simulink model "testPacketSend"  (R2014a)
settings: Solver=FixedStepDiscrete  StartTime=0.0  StopTime=Inf  FixedStep=0.001  RelTol=1e-3
InitFcn:
  | testSerializedParams_Initialize();
undefined symbols (not defined in the file or in its folder): macaddr
libraries: xpcnetworkbufferlib x1, xpcethernetlib x1, libButtons x1, libBusSerialize x1
settings Model: xpc_rtwmakecfg_data=_xpcnblib__xpcetherlib__xpcether8255xlib__xpcetherGbElib_  SimulationMode=external  BufferReuse=off  Creator=shenoylab  LastModifiedBy=shenoylab
settings SolverCC: EnableConcurrentExecution=on
settings DataIOCC: SignalLoggingSaveFormat=ModelDataLogs
settings OptimizationCC: BlockReduction=off  OptimizeBlockIOStorage=off  BufferReuse=off  GlobalBufferReuse=off  ExpressionFolding=off  LocalBlockOutputs=off
settings DebuggingCC: SaveWithDisabledLinksMsg=none  MultiTaskDSMMsg=warning  MultiTaskCondExecSysMsg=none  StateNameClashWarn=warning
settings HardwareCC: ProdIntDivRoundTo=Zero  ProdEndianess=LittleEndian  ProdHWDeviceType=Generic->32-bit x86 compatible
settings RTWCC: SystemTargetFile=slrt.tlc  TemplateMakefile=slrt_default_tmf  Description=Simulink Real-Time  GenerateReport=on  ProcessScript=slrt_make_rtw_hook  LaunchReport=on  IncludeERTFirstTime=on  RTWCompilerOptimization=On
settings CodeAppCC: MATLABSourceComments=on
settings SimulinkRealTimeCC: GeneratePreprocessorConditionals=Disable all  EnableShiftOperators=on  xpcDblBuff=on

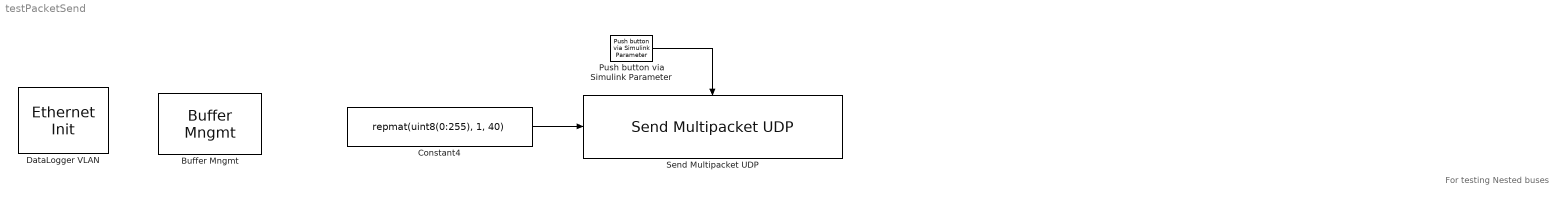
== system testPacketSend ==
  note: For testing Nested buses
  "Buffer Mngmt " : xpcnetworkbufferlib/Buffer Mngmt   Priority=-1  SampleTime=-1  PoolSizes=[256 512 1024 2048]  ShowTune=off
  Constant4 : Constant  Value=repmat(uint8(0:255), 1, 40)
  DataLogger VLAN : xpcethernetlib/Ethernet Init   Priority=-1  ID=2  Driver=Intel 8255x  Bus=3  Slot=5  SampleTime=-1  AddressSource=EEPROM  MAC=macaddr('00:00:00:00:00:00')  TxSA=off  RxPromiscuous=off  Multicast={}  RxBad=off  RxShort=off  MaxMTU=1518  TxThreshold=224  TxBuffers=256  RxBuffers=64  ShowTune=off  NumRxBlks=1
  Push button via Simulink Parameter : libButtons/Push button via Simulink Parameter  paramName='paramtestSerializedParamsExtern0x2FPushButtonViaSimulinkParamet'  Ts=0.001
  Send Multipacket UDP : libBusSerialize/Send Multipacket UDP  transmitId=2  sourceIP=[192 168 1 1]  sourcePort=20000  destIP=[192 168 1 255]  destPort=25000  destMac=macaddr('ff:ff:ff:ff:ff:ff')  ID=2  prependHeader=off
  wires:
  Push button via Simulink Parameter/1 -> Send Multipacket UDP/Enable
  Constant4/1 -> Send Multipacket UDP/1
